simulink model "inverter180degree"  (R2025a)
settings: Solver=VariableStepAuto  StartTime=0.0  StopTime=10.0  RelTol=1e-3
libraries: spsMosfetLib x6, spsSeriesRLCBranchLib x3, spsVoltageMeasurementLib x3, spsDCVoltageSourceLib x1, sps_lib x1
settings Model: Creator=gades  LastModifiedBy=gades

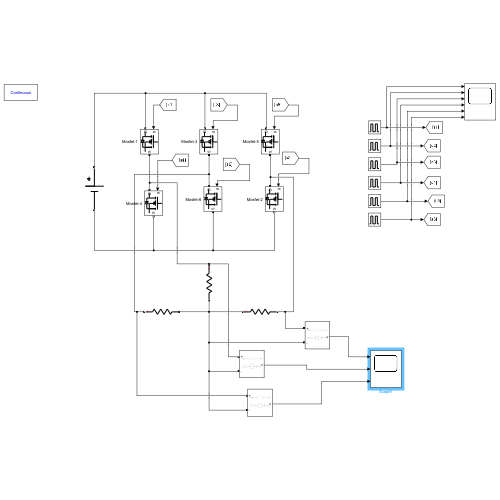
[thumbnail: Simulink's stored preview of the top-level diagram]
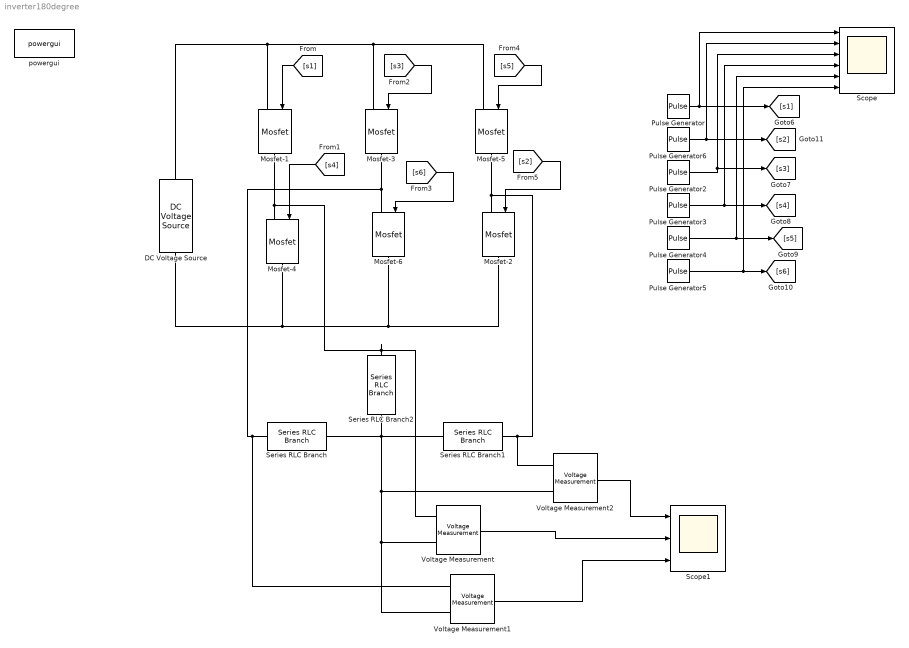
== system inverter180degree ==
  DC Voltage Source : spsDCVoltageSourceLib/DC Voltage Source  Amplitude=230  Measurements=None
  Mosfet-{1..6} (6 alike) : spsMosfetLib/Mosfet  Ron=0.1  Lon=0  Rd=0.01  Vfd=0  IC=0  Rs=1e5  Cs=inf  Measurements=off
  Pulse Generator : DiscretePulseGenerator  PulseType=Time based  Period=0.1  PulseWidth=50
  Pulse Generator2 : DiscretePulseGenerator  PulseType=Time based  Period=0.1  PulseWidth=50  PhaseDelay=0.1/3
  Pulse Generator3 : DiscretePulseGenerator  PulseType=Time based  Period=0.1  PulseWidth=50  PhaseDelay=0.1/2
  Pulse Generator4 : DiscretePulseGenerator  PulseType=Time based  Period=0.1  PulseWidth=50  PhaseDelay=0.2/3
  Pulse Generator5 : DiscretePulseGenerator  PulseType=Time based  Period=0.1  PulseWidth=50  PhaseDelay=0.5/6
  Pulse Generator6 : DiscretePulseGenerator  PulseType=Time based  Period=0.1  PulseWidth=50  PhaseDelay=0.1/6
  Scope : Scope  NumInputPorts=6
      settings: ActiveDisplayYMinimum=-0.12499999999999997  ActiveDisplayYMaximum=1.125
  Scope1 : Scope  NumInputPorts=3
      settings: ActiveDisplayYMinimum=-189.76860111828162  ActiveDisplayYMaximum=189.76860111828159
  Series RLC Branch : spsSeriesRLCBranchLib/Series RLC Branch  LConnTagsString=__new0  RConnTagsString=__new0  BranchType=R  Resistance=10  Inductance=1e-3  SetiL0=off  InitialCurrent=0  Capacitance=1e-6  Setx0=off  InitialVoltage=0  Measurements=None
  Series RLC Branch1 : spsSeriesRLCBranchLib/Series RLC Branch  LConnTagsString=__new0  RConnTagsString=__new0  BranchType=R  Resistance=10  Inductance=1e-3  SetiL0=off  InitialCurrent=0  Capacitance=1e-6  Setx0=off  InitialVoltage=0  Measurements=None
  Series RLC Branch2 : spsSeriesRLCBranchLib/Series RLC Branch  LConnTagsString=__new0  RConnTagsString=__new0  BranchType=R  Resistance=10  Inductance=1e-3  SetiL0=off  InitialCurrent=0  Capacitance=1e-6  Setx0=off  InitialVoltage=0  Measurements=None
  Voltage Measurement : spsVoltageMeasurementLib/Voltage Measurement  PhasorSimulation=off  OutputType=Complex  PSBequivalent=0
  Voltage Measurement1 : spsVoltageMeasurementLib/Voltage Measurement  PhasorSimulation=off  OutputType=Complex  PSBequivalent=0
  Voltage Measurement2 : spsVoltageMeasurementLib/Voltage Measurement  PhasorSimulation=off  OutputType=Complex  PSBequivalent=0
  powergui : sps_lib/powergui  Priority=1  SimulationMode=Continuous  SampleTime=50e-6  frequency=60  Iterations=50  frequencyindice=0  Pbase=100e6  ErrMax=1e-4  UnitsV=kV  UnitsW=MW  buscounter=0  FunctionMessages=off  echomessages=off  EnableUseOfTLC=off  CurrentSourceSwitches=off  DisableSnubberDevices=off  DisableRonSwitches=off  DisableVfSwitches=off  DisplayEquations=off  AutomaticDiscreteSolvers=off  SolverType=Tustin/Backward Euler (TBE)  Interpol=off  ExternalGateDelay=off  methode=off  Ts=100  x0status=blocks  SPID=on  SwTol=0  HookPort=off  NonlinearTolerance=1e-4  nMaxIteration=100  ContinueOnMaxIteration=off  RestoreLinks=warning  ResistiveCurrentMeasurement=off  Frange=[0:2:500]  Ylog=off  Xlog=on  ShowGrid=off  save=off  variable=ZData  structure=0  ZoomFFT=off  StartTime=0.0  cycles=1  DisplayStyle=1  fundamental=60  FreqAxis=off  MaxFrequency=1000  frequencyindicesteady=1  RmsSteady=1  display=off
  wires:
  [s1] -> Mosfet-1/1
  [s4] -> Mosfet-4/1
  [s3] -> Mosfet-3/1
  [s6] -> Mosfet-6/1
  [s5] -> Mosfet-5/1
  [s2] -> Mosfet-2/1
  Pulse Generator/1 -> Scope/1, [s1]
  Pulse Generator6/1 -> Scope/2, [s2]
  Pulse Generator2/1 -> Scope/3, [s3]
  Pulse Generator3/1 -> Scope/4, [s4]
  Pulse Generator4/1 -> Scope/5, [s5]
  Pulse Generator5/1 -> Scope/6, [s6]
  Voltage Measurement2/1 -> Scope1/1
  Voltage Measurement/1 -> Scope1/2
  Voltage Measurement1/1 -> Scope1/3
  connections:
  Mosfet-2/LConn1 -- Voltage Measurement2/LConn1 -- Series RLC Branch1/RConn1 -- Mosfet-5/RConn1
  Mosfet-6/LConn1 -- Voltage Measurement1/LConn1 -- Series RLC Branch/LConn1 -- Mosfet-3/RConn1
  DC Voltage Source/RConn1 -- Mosfet-5/LConn1 -- Mosfet-3/LConn1 -- Mosfet-1/LConn1
  DC Voltage Source/LConn1 -- Mosfet-2/RConn1 -- Mosfet-6/RConn1 -- Mosfet-4/RConn1
  Series RLC Branch1/LConn1 -- Voltage Measurement1/LConn2 -- Voltage Measurement/LConn2 -- Voltage Measurement2/LConn2 -- Series RLC Branch2/RConn1 -- Series RLC Branch/RConn1
  Mosfet-1/RConn1 -- Voltage Measurement/LConn1 -- Series RLC Branch2/LConn1 -- Mosfet-4/LConn1
